simulink model "planta_perturbacion"  (R2018a)
settings: Solver=VariableStepAuto  StartTime=0.0  StopTime=600  RelTol=1e-3
values from neighbouring files (symbols this model uses):
  we = 0.3    [evaluar_rechazo_perturbacion.m]
  wn = 0.3    [evaluar_rechazo_perturbacion.m]
  xi = 0.01    [evaluar_rechazo_perturbacion.m]
libraries: simulink x1
settings Model: Creator=pablo  LastModifiedBy=pablo

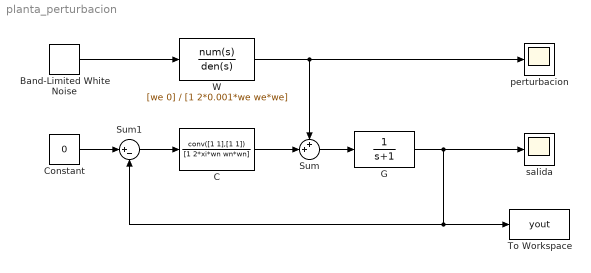
== system planta_perturbacion ==
  Band-Limited White Noise : simulink/Sources/Band-Limited White Noise  Cov=[1]  Ts=0.1  seed=[23341]
  C : TransferFcn  Numerator=conv([1 1],[1 1])  Denominator=[1 2*xi*wn wn*wn]
  Constant : Constant  Value=0
  G : TransferFcn  Denominator=[1 1]
  Sum : Sum  Inputs=++|
  Sum1 : Sum  Inputs=|+-
  To Workspace : ToWorkspace  VariableName=yout  SaveFormat=Timeseries  SampleTime=-1
  W : TransferFcn  Numerator=[we 0]  Denominator=[1 2*0.001*we we*we]
  perturbacion : Scope
  salida : Scope
  wires:
  G/1 -> Sum1/2, To Workspace/1, salida/1
  Sum/1 -> G/1
  C/1 -> Sum/2
  Band-Limited White Noise/1 -> W/1
  W/1 -> perturbacion/1, Sum/1
  Sum1/1 -> C/1
  Constant/1 -> Sum1/1
